simulink model "TP1P06"  (R2017a)
settings: Solver=FixedStepAuto  StartTime=0.0  StopTime=10.0  FixedStep=0.05  RelTol=1e-3
values from neighbouring files (symbols this model uses):
  g = 9.81    [calcul_K.m]
undefined symbols (not defined in the file or in its folder): alpha0, l, v0
libraries: simulink x1
settings Model: Creator=rxambili  LastModifiedBy=rxambili

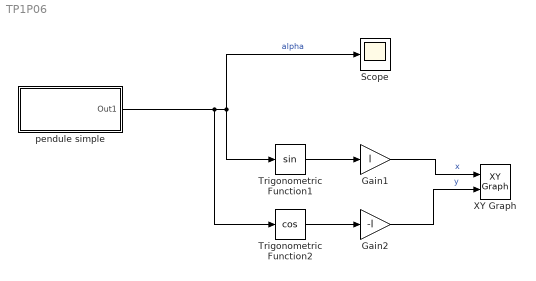
== system TP1P06 ==
  Gain1 : Gain  Gain=l
  Gain2 : Gain  Gain=-l
  Scope : Scope
  Trigonometric Function1 : Trigonometry
  Trigonometric Function2 : Trigonometry  Operator=cos
  XY Graph : simulink/Sinks/XY Graph  xmin=-2  xmax=2  ymin=-2  ymax=2  st=-1
  "pendule simple " : Subsystem
  wires:
  Gain1/1 -> XY Graph/1  "x"
  Trigonometric Function2/1 -> Gain2/1
  Trigonometric Function1/1 -> Gain1/1
  "pendule simple "/1(Out1) -> Trigonometric Function2/1, Trigonometric Function1/1, Scope/1  "alpha"
  Gain2/1 -> XY Graph/2  "y"

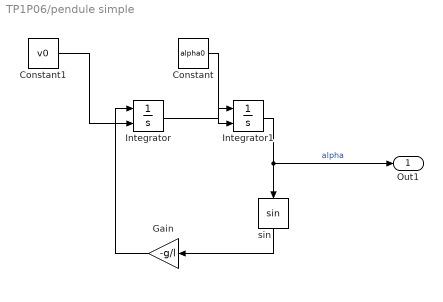
== system TP1P06/pendule simple  ==
  Constant : Constant  Value=alpha0
  Constant1 : Constant  Value=v0
  Gain : Gain  Gain=-g/l
  Integrator : Integrator  InitialConditionSource=external
  Integrator1 : Integrator  InitialConditionSource=external  InitialCondition=alpha0
  sin : Trigonometry
  Out1 : Outport
  wires:
  Constant/1 -> Integrator1/2
  sin/1 -> Gain/1
  Integrator/1 -> Integrator1/1
  Integrator1/1 -> Out1/1, sin/1  "alpha"
  Gain/1 -> Integrator/1
  Constant1/1 -> Integrator/2
